simulink model "HLS_VMC_testing"  (R2025a)
settings: Solver=VariableStepAuto  StartTime=0.0  StopTime=0.0001  RelTol=1e-3
InitFcn:
  | fs = 500e6;
values from neighbouring files (symbols this model uses):
  N = length(X)    [outputPlots.m]
undefined symbols (not defined in the file or in its folder): A, es1, i, S, vsva2488, xcvr1602
libraries: hdlBasic x98, hlsBasic x64, aieUtilities x18, dspsrcs4 x15, dspxfrm3 x2, hdlDSPIP x2, hlsUtilities x1, vmcUtilities x1
(part 4 of 4)

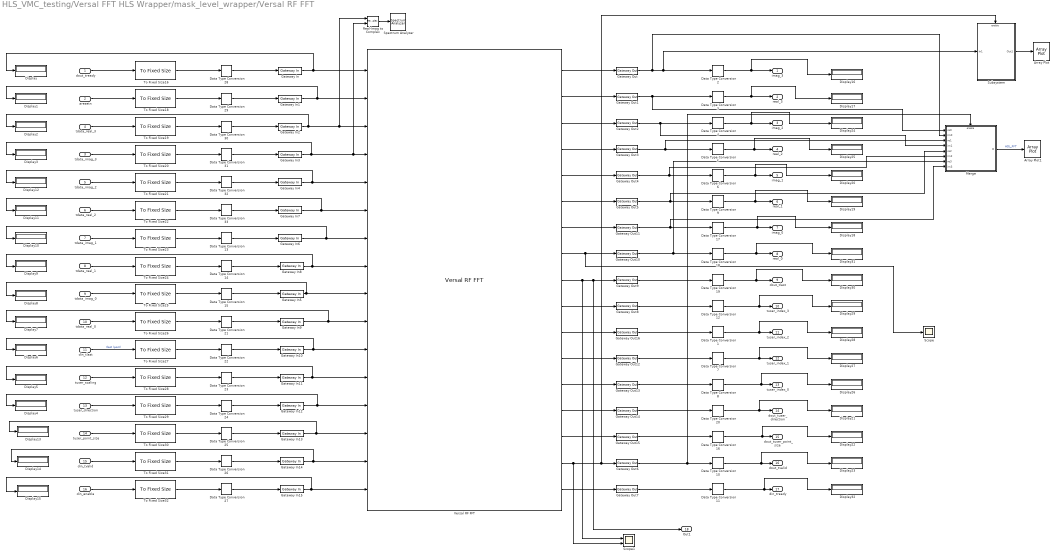
== system HLS_VMC_testing/Versal FFT HLS Wrapper/mask_level_wrapper/Versal RF FFT ==
  dout_tready : Inport
  aresetn : Inport  Port=2
  tdata_imag_3 : Inport  Port=3
  tdata_real_3 : Inport  Port=4
  tdata_imag_2 : Inport  Port=5
  tdata_real_2 : Inport  Port=6
  tdata_imag_1 : Inport  Port=7
  tdata_real_1 : Inport  Port=8
  tdata_imag_0 : Inport  Port=9
  tdata_real_0 : Inport  Port=10
  din_tlast : Inport  Port=11
  tuser_scaling : Inport  Port=12
  tuser_direction : Inport  Port=13
  tuser_point_size : Inport  Port=14
  din_tvalid : Inport  Port=15
  din_enable : Inport  Port=16
  Array Plot : ArrayPlot  WindowPosition=[880.000000,470.000000,800.000000,500.000000,]  ScopeFrameLocation=window  YLimits=[-10 10]
  Array Plot1 : ArrayPlot  WindowPosition=[880.000000,470.000000,800.000000,500.000000,]  ScopeFrameLocation=window  YLimits=[-10 10]
  Data Type Conversion{1,7..8,12} (4 alike) : hlsBasic/Data Type Conversion  OutDataType=data type expression  TypeExp='x_ufix12'  Signedness=Signed  WordLength=16  FractionalLength=0  RoundingMode=Truncation to minus infinity  OverflowMode=Wrap around
  Data Type Conversion{10..11,19..20} (4 alike) : hlsBasic/Data Type Conversion  OutDataType=data type expression  TypeExp='x_ufix1'  Signedness=Signed  WordLength=16  FractionalLength=0  RoundingMode=Truncation to minus infinity  OverflowMode=Wrap around
  Data Type Conversion{13..15,21..33} (16 alike) : hlsBasic/Data Type Conversion  OutDataType=double  TypeExp=''  Signedness=Signed  WordLength=16  FractionalLength=0  RoundingMode=Truncation to minus infinity  OverflowMode=Wrap around
  Data Type Conversion16 : hlsBasic/Data Type Conversion  OutDataType=data type expression  TypeExp='x_ufix4'  Signedness=Signed  WordLength=16  FractionalLength=0  RoundingMode=Truncation to minus infinity  OverflowMode=Wrap around
  Data Type Conversion{2..6,9,17..18} (8 alike) : hlsBasic/Data Type Conversion  OutDataType=data type expression  TypeExp='x_sfix16_En15'  Signedness=Signed  WordLength=16  FractionalLength=0  RoundingMode=Truncation to minus infinity  OverflowMode=Wrap around
  Display{,1..32} (33 alike) : Display
  Gateway In : hdlBasic/Gateway In  gui_display_data_type=Boolean  arith_type=Boolean  n_bits=16  bin_pt=15  preci_type=Single  exp_width=8  frac_width=24  rows=1  columns=1  quantization="Round  (unbiased: +/- Inf)"  overflow=Saturate  period=1/fs  UseAsADC=off  ADCChannel='1'  interface=None  automatic_assignment=on  address_offset=hex2dec('00')  intf_name=''  intf_description=''  default_value=0  timing_constraint=None  locs_specified=off  LOCs={}  io_standard={}  inherit_from_input=off  hdl_port=on  XmcBlockStatus=1  maskContainerNames=group4  block_type=gatewayin  block_config=sysgen:gateway_in_config  block_width_w=590  block_height_w=620  block_width=640  block_height=850
  Gateway In{1,10,14..15} (4 alike) : hdlBasic/Gateway In  gui_display_data_type=Boolean  arith_type=Boolean  n_bits=16  bin_pt=14  preci_type=Single  exp_width=8  frac_width=24  rows=1  columns=1  quantization="Round  (unbiased: +/- Inf)"  overflow=Saturate  period=1/fs  UseAsADC=off  ADCChannel='1'  interface=None  automatic_assignment=on  address_offset=hex2dec('00')  intf_name=''  intf_description=''  default_value=0  timing_constraint=None  locs_specified=off  LOCs={}  io_standard={}  inherit_from_input=off  hdl_port=on  XmcBlockStatus=1  maskContainerNames=group4  block_type=gatewayin  block_config=sysgen:gateway_in_config  block_width_w=590  block_height_w=620  block_width=640  block_height=850
  Gateway In11 : hdlBasic/Gateway In  gui_display_data_type=Fixed-point  arith_type=Unsigned  n_bits=13  bin_pt=13  preci_type=Single  exp_width=8  frac_width=24  rows=1  columns=1  quantization="Round  (unbiased: +/- Inf)"  overflow=Saturate  period=1/fs  UseAsADC=off  ADCChannel='1'  interface=None  automatic_assignment=on  address_offset=hex2dec('00')  intf_name=''  intf_description=''  default_value=0  timing_constraint=None  locs_specified=off  LOCs={}  io_standard={}  inherit_from_input=off  hdl_port=on  XmcBlockStatus=1  maskContainerNames=group4  block_type=gatewayin  block_config=sysgen:gateway_in_config  block_width_w=590  block_height_w=620  block_width=640  block_height=850
  Gateway In12 : hdlBasic/Gateway In  gui_display_data_type=Fixed-point  arith_type=Unsigned  n_bits=1  bin_pt=0  preci_type=Single  exp_width=8  frac_width=24  rows=1  columns=1  quantization="Round  (unbiased: +/- Inf)"  overflow=Saturate  period=1/fs  UseAsADC=off  ADCChannel='1'  interface=None  automatic_assignment=on  address_offset=hex2dec('00')  intf_name=''  intf_description=''  default_value=0  timing_constraint=None  locs_specified=off  LOCs={}  io_standard={}  inherit_from_input=off  hdl_port=on  XmcBlockStatus=1  maskContainerNames=group4  block_type=gatewayin  block_config=sysgen:gateway_in_config  block_width_w=590  block_height_w=620  block_width=640  block_height=850
  Gateway In13 : hdlBasic/Gateway In  gui_display_data_type=Fixed-point  arith_type=Unsigned  n_bits=4  bin_pt=0  preci_type=Single  exp_width=8  frac_width=24  rows=1  columns=1  quantization="Round  (unbiased: +/- Inf)"  overflow=Saturate  period=1/fs  UseAsADC=off  ADCChannel='1'  interface=None  automatic_assignment=on  address_offset=hex2dec('00')  intf_name=''  intf_description=''  default_value=0  timing_constraint=None  locs_specified=off  LOCs={}  io_standard={}  inherit_from_input=off  hdl_port=on  XmcBlockStatus=1  maskContainerNames=group4  block_type=gatewayin  block_config=sysgen:gateway_in_config  block_width_w=590  block_height_w=620  block_width=640  block_height=850
  Gateway In{2..9} (8 alike) : hdlBasic/Gateway In  gui_display_data_type=Fixed-point  arith_type=Signed (2's comp)  n_bits=18  bin_pt=17  preci_type=Single  exp_width=8  frac_width=24  rows=1  columns=1  quantization="Round  (unbiased: +/- Inf)"  overflow=Saturate  period=1/fs  UseAsADC=off  ADCChannel='1'  interface=None  automatic_assignment=on  address_offset=hex2dec('00')  intf_name=''  intf_description=''  default_value=0  timing_constraint=None  locs_specified=off  LOCs={}  io_standard={}  inherit_from_input=off  hdl_port=on  XmcBlockStatus=1  maskContainerNames=group4  block_type=gatewayin  block_config=sysgen:gateway_in_config  block_width_w=590  block_height_w=620  block_width=640  block_height=850
  Gateway Out{,1..16} (17 alike) : hdlBasic/Gateway Out  inherit_from_input=off  bool_to_boolean=off  hdl_port=on  rows=1  columns=1  UseAsDAC=off  DACChannel='1'  interface=None  automatic_assignment=on  address_offset=hex2dec('00')  intf_name=''  intf_description=''  timing_constraint=None  locs_specified=off  LOCs={}  io_standard={}  XmcBlockStatus=1  maskContainerNames=group4  block_type=gatewayout  block_config=sysgen:gateway_out_config  block_width_w=590  block_height_w=620  block_width=620  block_height=750
  Merge : Subsystem
  Real-Imag to Complex : RealImagToComplex
  Scope : Scope
      settings: ActiveDisplayYMinimum=-1  ActiveDisplayYMaximum=1  DataLoggingVariableName=ScopeData10
  Scope1 : Scope  NumInputPorts=2
      settings: ActiveDisplayYMinimum=-1  ActiveDisplayYMaximum=1  DataLoggingVariableName=ScopeData9
  Spectrum Analyzer : SpectrumAnalyzer  WindowPosition=[591.000000,490.000000,800.000000,500.000000,]  ScopeFrameLocation=window  WindowInvariantSamplesPerUpdate=on  YLimits=[-31.4263 39.9556]
  Subsystem : Subsystem
  To Fixed Size{16,18..32} (16 alike) : aieUtilities/To Fixed Size  Mode=Stop simulation when input variable-size signal is not full  OutputSize=Inherit: Same as input  CopyMethod=Buffer samples to form output  HasStatusOutput=on
  Versal RF FFT : hdlDSPIP/Versal RF FFT  sample_rate=4  fft_max_point_size_temp=1024  fft_max_point_size=10  fft_scaling=on  fft_reorder=on  events=off  ip_name=Versal RF FFT  enable_all_ports=false  mode=Streaming FFT  ip_version=1.1  dsptool_ready=false  ipcore_usecache=true  ipcore_useipmodelcache=true  wrapper_available=true  port_translation_map={ 'S_AXIS_aclken' => 'en', 'aresetn' => 'rst' }  structural_sim=true  ipcore_do_not_force_period=true  XmcBlockStatus=1  maskContainerNames=tabcontainer1  block_type=vrf_fft_v1_0  block_config=sysgen:rodinimport_config
  imag_3 : Outport
  real_3 : Outport  Port=2
  imag_2 : Outport  Port=3
  real_2 : Outport  Port=4
  imag_1 : Outport  Port=5
  real_1 : Outport  Port=6
  imag_0 : Outport  Port=7
  real_0 : Outport  Port=8
  dout_tlast : Outport  Port=9
  tuser_index_3 : Outport  Port=10
  tuser_index_2 : Outport  Port=11
  tuser_index_1 : Outport  Port=12
  tuser_index_0 : Outport  Port=13
  dout_tuser_direction : Outport  Port=14
  dout_tuser_point_size : Outport  Port=15
  dout_tvalid : Outport  Port=16
  din_tready : Outport  Port=17
  Out1 : Outport  Port=18
  wires:
  dout_tready/1 -> To Fixed Size16/1
  aresetn/1 -> To Fixed Size18/1
  tuser_point_size/1 -> To Fixed Size30/1
  tuser_direction/1 -> To Fixed Size29/1
  tuser_scaling/1 -> To Fixed Size28/1
  din_tlast/1 -> To Fixed Size27/1  "tlast (post)"
  din_tvalid/1 -> To Fixed Size31/1
  tdata_real_3/1 -> To Fixed Size19/1
  tdata_real_0/1 -> To Fixed Size26/1
  tdata_real_2/1 -> To Fixed Size22/1
  tdata_real_1/1 -> To Fixed Size24/1
  tdata_imag_0/1 -> To Fixed Size25/1
  tdata_imag_1/1 -> To Fixed Size23/1
  tdata_imag_2/1 -> To Fixed Size21/1
  tdata_imag_3/1 -> To Fixed Size20/1
  din_enable/1 -> To Fixed Size32/1
  Versal RF FFT/2 -> Gateway Out1/1
  Versal RF FFT/3 -> Gateway Out2/1
  Versal RF FFT/4 -> Gateway Out3/1
  Versal RF FFT/5 -> Gateway Out4/1
  Versal RF FFT/6 -> Gateway Out5/1
  Versal RF FFT/7 -> Gateway Out11/1
  Versal RF FFT/8 -> Scope/1, Gateway Out10/1
  Versal RF FFT/10 -> Gateway Out8/1
  Versal RF FFT/11 -> Gateway Out16/1
  Versal RF FFT/1 -> Gateway Out/1
  To Fixed Size16/1 -> Data Type Conversion28/1
  To Fixed Size18/1 -> Data Type Conversion29/1
  To Fixed Size19/1 -> Data Type Conversion30/1
  To Fixed Size20/1 -> Data Type Conversion31/1
  To Fixed Size21/1 -> Data Type Conversion32/1
  To Fixed Size22/1 -> Data Type Conversion33/1
  To Fixed Size23/1 -> Data Type Conversion13/1
  To Fixed Size24/1 -> Data Type Conversion14/1
  To Fixed Size25/1 -> Data Type Conversion15/1
  To Fixed Size26/1 -> Data Type Conversion21/1
  To Fixed Size27/1 -> Data Type Conversion22/1
  To Fixed Size28/1 -> Data Type Conversion23/1
  To Fixed Size29/1 -> Data Type Conversion24/1
  To Fixed Size30/1 -> Data Type Conversion25/1
  To Fixed Size31/1 -> Data Type Conversion26/1
  To Fixed Size32/1 -> Data Type Conversion27/1
  Gateway In/1 -> Display/1, Versal RF FFT/1
  Gateway In1/1 -> Display1/1, Versal RF FFT/2
  Gateway In4/1 -> Display12/1, Versal RF FFT/5
  Gateway In7/1 -> Display11/1, Versal RF FFT/6
  Gateway In6/1 -> Display10/1, Versal RF FFT/7
  Gateway In9/1 -> Display7/1, Versal RF FFT/10
  Gateway In5/1 -> Display8/1, Versal RF FFT/9
  Gateway In10/1 -> Display6/1, Versal RF FFT/11
  Gateway In11/1 -> Display5/1, Versal RF FFT/12
  Gateway Out1/1 -> Merge/1(re0), Data Type Conversion3/1
  Gateway Out2/1 -> Merge/4(im1), Data Type Conversion4/1
  Gateway Out3/1 -> Merge/3(re1), Data Type Conversion5/1
  Gateway Out4/1 -> Merge/6(im2), Data Type Conversion6/1
  Gateway Out5/1 -> Merge/5(re2), Data Type Conversion9/1
  Gateway Out11/1 -> Merge/8(im3), Data Type Conversion17/1
  Gateway Out10/1 -> Merge/7(re3), Data Type Conversion18/1
  Gateway Out9/1 -> Data Type Conversion19/1
  Gateway Out6/1 -> Merge/Enable, Data Type Conversion10/1
  Gateway Out7/1 -> Data Type Conversion11/1
  Gateway Out8/1 -> Data Type Conversion12/1
  Gateway Out16/1 -> Data Type Conversion1/1
  Gateway Out12/1 -> Data Type Conversion7/1
  Gateway Out13/1 -> Data Type Conversion8/1
  Gateway Out15/1 -> Data Type Conversion16/1
  Gateway Out14/1 -> Data Type Conversion20/1
  Data Type Conversion2/1 -> Display16/1, imag_3/1
  Data Type Conversion3/1 -> Display17/1, real_3/1
  Data Type Conversion4/1 -> Display24/1, imag_2/1
  Data Type Conversion5/1 -> Display25/1, real_2/1
  Data Type Conversion6/1 -> Display20/1, imag_1/1
  Data Type Conversion9/1 -> Display19/1, real_1/1
  Data Type Conversion17/1 -> Display18/1, imag_0/1
  Data Type Conversion19/1 -> Display30/1, dout_tlast/1
  Data Type Conversion12/1 -> Display29/1, tuser_index_3/1
  Data Type Conversion1/1 -> Display28/1, tuser_index_2/1
  Data Type Conversion7/1 -> Display27/1, tuser_index_1/1
  Data Type Conversion8/1 -> Display26/1, tuser_index_0/1
  Data Type Conversion20/1 -> Display21/1, dout_tuser_direction/1
  Data Type Conversion16/1 -> Display22/1, dout_tuser_point_size/1
  Data Type Conversion10/1 -> Display23/1, dout_tvalid/1
  Data Type Conversion11/1 -> Display32/1, din_tready/1
  Versal RF FFT/9 -> Scope1/1, Out1/1, Gateway Out9/1
  Gateway In12/1 -> Display4/1, Versal RF FFT/13
  Gateway In14/1 -> Display14/1, Versal RF FFT/15
  Gateway In15/1 -> Display15/1, Versal RF FFT/16
  Gateway In13/1 -> Display13/1, Versal RF FFT/14
  Versal RF FFT/12 -> Gateway Out12/1
  Versal RF FFT/13 -> Gateway Out13/1
  Versal RF FFT/14 -> Gateway Out14/1
  Versal RF FFT/15 -> Gateway Out15/1
  Versal RF FFT/16 -> Scope1/2, Subsystem/Enable, Gateway Out6/1
  Versal RF FFT/17 -> Gateway Out7/1
  Data Type Conversion28/1 -> Gateway In/1
  Data Type Conversion29/1 -> Gateway In1/1
  Data Type Conversion30/1 -> Gateway In2/1
  Data Type Conversion31/1 -> Gateway In3/1
  Data Type Conversion32/1 -> Gateway In4/1
  Data Type Conversion33/1 -> Gateway In7/1
  Data Type Conversion13/1 -> Gateway In6/1
  Data Type Conversion14/1 -> Gateway In8/1
  Data Type Conversion15/1 -> Gateway In5/1
  Data Type Conversion21/1 -> Gateway In9/1
  Data Type Conversion22/1 -> Gateway In10/1
  Data Type Conversion23/1 -> Gateway In11/1
  Data Type Conversion24/1 -> Gateway In12/1
  Data Type Conversion25/1 -> Gateway In13/1
  Data Type Conversion26/1 -> Gateway In14/1
  Data Type Conversion27/1 -> Gateway In15/1
  Gateway In8/1 -> Display9/1, Versal RF FFT/8
  Data Type Conversion18/1 -> Display31/1, real_0/1
  Gateway In2/1 -> Display2/1, Real-Imag to Complex/1, Versal RF FFT/3
  Gateway In3/1 -> Display3/1, Real-Imag to Complex/2, Versal RF FFT/4
  Real-Imag to Complex/1 -> Spectrum Analyzer/1
  Gateway Out/1 -> Merge/2(im0), Subsystem/1(In1), Data Type Conversion2/1
  Subsystem/1(Out1) -> Array Plot/1
  Merge/1(O) -> Array Plot1/1  "HDL_FFT"

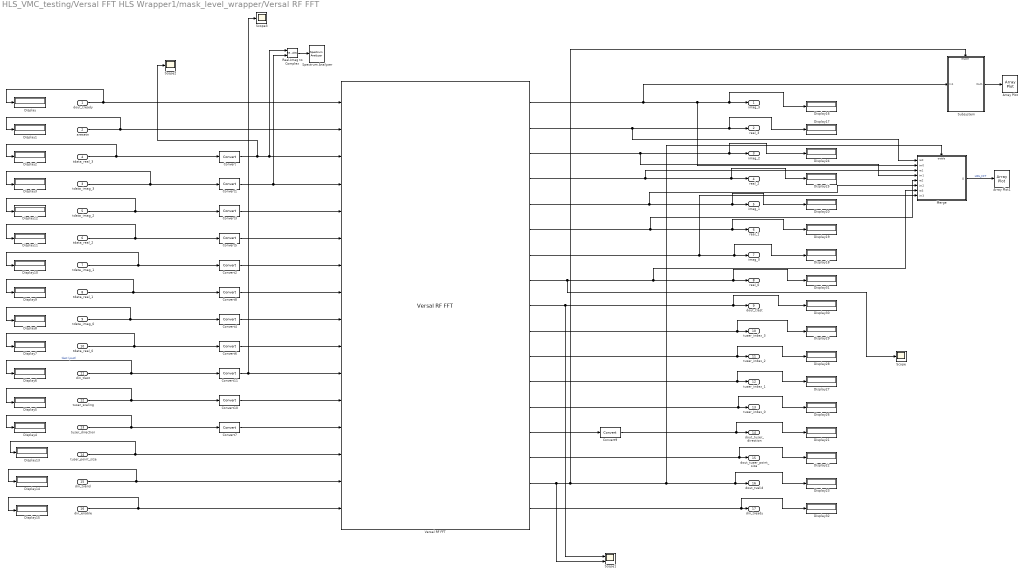
== system HLS_VMC_testing/Versal FFT HLS Wrapper1/mask_level_wrapper/Versal RF FFT ==
  dout_tready : Inport
  aresetn : Inport  Port=2
  tdata_imag_3 : Inport  Port=3
  tdata_real_3 : Inport  Port=4
  tdata_imag_2 : Inport  Port=5
  tdata_real_2 : Inport  Port=6
  tdata_imag_1 : Inport  Port=7
  tdata_real_1 : Inport  Port=8
  tdata_imag_0 : Inport  Port=9
  tdata_real_0 : Inport  Port=10
  din_tlast : Inport  Port=11
  tuser_scaling : Inport  Port=12
  tuser_direction : Inport  Port=13
  tuser_point_size : Inport  Port=14
  din_tvalid : Inport  Port=15
  din_enable : Inport  Port=16
  Array Plot : ArrayPlot  WindowPosition=[1.000000,1.000000,2560.000000,1389.000000,]  ScopeFrameLocation=window  YLimits=[-10 10]
  Array Plot1 : ArrayPlot  WindowPosition=[1.000000,1.000000,2560.000000,1389.000000,]  ScopeFrameLocation=window  YLimits=[-10 10]
  Convert{,1..6,8} (8 alike) : hdlBasic/Convert  gui_display_data_type=Fixed-point  arith_type="Signed  (2's comp)"  n_bits=18  bin_pt=17  float_type=Single  exp_bits=8  fraction_bits=24  quantization=Truncate  overflow=Wrap  en=off  latency=0  pipeline=off  XmcBlockStatus=1  maskContainerNames=group2  block_type=convert  block_config=sysgen:Convert_config  block_width=595  block_height=885
  Convert10 : hdlBasic/Convert  gui_display_data_type=Fixed-point  arith_type=Unsigned  n_bits=13  bin_pt=13  float_type=Single  exp_bits=8  fraction_bits=24  quantization=Truncate  overflow=Wrap  en=off  latency=0  pipeline=off  XmcBlockStatus=1  maskContainerNames=group2  block_type=convert  block_config=sysgen:Convert_config  block_width=595  block_height=885
  Convert11 : hdlBasic/Convert  gui_display_data_type=Boolean  arith_type=Boolean  n_bits=18  bin_pt=17  float_type=Single  exp_bits=8  fraction_bits=24  quantization=Truncate  overflow=Wrap  en=off  latency=0  pipeline=off  XmcBlockStatus=1  maskContainerNames=group2  block_type=convert  block_config=sysgen:Convert_config  block_width=595  block_height=885
  Convert7 : hdlBasic/Convert  gui_display_data_type=Fixed-point  arith_type=Unsigned  n_bits=1  bin_pt=0  float_type=Single  exp_bits=8  fraction_bits=24  quantization=Truncate  overflow=Wrap  en=off  latency=0  pipeline=off  XmcBlockStatus=1  maskContainerNames=group2  block_type=convert  block_config=sysgen:Convert_config  block_width=595  block_height=885
  Convert9 : hdlBasic/Convert  gui_display_data_type=Boolean  arith_type=Boolean  n_bits=1  bin_pt=0  float_type=Single  exp_bits=8  fraction_bits=24  quantization=Truncate  overflow=Wrap  en=off  latency=0  pipeline=off  XmcBlockStatus=1  maskContainerNames=group2  block_type=convert  block_config=sysgen:Convert_config  block_width=595  block_height=885
  Display{,1..32} (33 alike) : Display
  Merge : Subsystem
  Real-Imag to Complex : RealImagToComplex
  Scope : Scope
      settings: ActiveDisplayYMinimum=-1  ActiveDisplayYMaximum=1  DataLoggingVariableName=ScopeData10
  Scope1 : Scope  NumInputPorts=2
      settings: ActiveDisplayYMinimum=-1  ActiveDisplayYMaximum=1  DataLoggingVariableName=ScopeData9
  Scope2 : Scope
      settings: ActiveDisplayYMinimum=-1  ActiveDisplayYMaximum=1  DataLoggingVariableName=ScopeData22
  Scope3 : Scope
      settings: ActiveDisplayYMinimum=-1  ActiveDisplayYMaximum=1  DataLoggingVariableName=ScopeData23
  Spectrum Analyzer : SpectrumAnalyzer  WindowPosition=[880.000000,470.000000,800.000000,500.000000,]  ScopeFrameLocation=window  WindowInvariantSamplesPerUpdate=on  Span=499999999.99999994  StartFrequency=-249999999.99999997  StopFrequency=249999999.99999997  YLimits=[-46.6022 38.4581]
  Subsystem : Subsystem
  Versal RF FFT : hdlDSPIP/Versal RF FFT  sample_rate=4  fft_max_point_size_temp=1024  fft_max_point_size=10  fft_scaling=on  fft_reorder=on  events=off  ip_name=Versal RF FFT  enable_all_ports=false  mode=Streaming FFT  ip_version=1.1  dsptool_ready=false  ipcore_usecache=true  ipcore_useipmodelcache=true  wrapper_available=true  port_translation_map={ 'S_AXIS_aclken' => 'en', 'aresetn' => 'rst' }  structural_sim=true  ipcore_do_not_force_period=true  XmcBlockStatus=1  maskContainerNames=tabcontainer1  block_type=vrf_fft_v1_0  block_config=sysgen:rodinimport_config
  imag_3 : Outport
  real_3 : Outport  Port=2
  imag_2 : Outport  Port=3
  real_2 : Outport  Port=4
  imag_1 : Outport  Port=5
  real_1 : Outport  Port=6
  imag_0 : Outport  Port=7
  real_0 : Outport  Port=8
  dout_tlast : Outport  Port=9
  tuser_index_3 : Outport  Port=10
  tuser_index_2 : Outport  Port=11
  tuser_index_1 : Outport  Port=12
  tuser_index_0 : Outport  Port=13
  dout_tuser_direction : Outport  Port=14
  dout_tuser_point_size : Outport  Port=15
  dout_tvalid : Outport  Port=16
  din_tready : Outport  Port=17
  wires:
  aresetn/1 -> Display1/1, Versal RF FFT/2
  din_tlast/1 -> Display6/1, Convert11/1  "tlast (post)"
  tdata_imag_2/1 -> Display12/1, Convert3/1
  tdata_imag_1/1 -> Display10/1, Convert2/1
  tdata_real_0/1 -> Display7/1, Convert6/1
  tdata_imag_0/1 -> Display8/1, Convert4/1
  Versal RF FFT/1 -> Merge/2(im0), Display16/1, imag_3/1, Subsystem/1(In1)
  Versal RF FFT/2 -> Display17/1, real_3/1, Merge/1(re0)
  Versal RF FFT/3 -> Display24/1, imag_2/1, Merge/4(im1)
  Versal RF FFT/4 -> Display25/1, real_2/1, Merge/3(re1)
  Versal RF FFT/5 -> Display20/1, imag_1/1, Merge/6(im2)
  Versal RF FFT/6 -> Display19/1, real_1/1, Merge/5(re2)
  Versal RF FFT/7 -> Display18/1, imag_0/1, Merge/8(im3)
  Versal RF FFT/9 -> Scope1/1, Display30/1, dout_tlast/1
  Versal RF FFT/10 -> Display29/1, tuser_index_3/1
  Versal RF FFT/11 -> Display28/1, tuser_index_2/1
  Versal RF FFT/12 -> Display27/1, tuser_index_1/1
  Versal RF FFT/13 -> Display26/1, tuser_index_0/1
  Versal RF FFT/14 -> Convert9/1
  Versal RF FFT/15 -> Display22/1, dout_tuser_point_size/1
  Versal RF FFT/16 -> Scope1/2, Merge/Enable, Display23/1, dout_tvalid/1, Subsystem/Enable
  Versal RF FFT/17 -> Display32/1, din_tready/1
  tdata_real_1/1 -> Display9/1, Convert8/1
  Versal RF FFT/8 -> Display31/1, real_0/1, Merge/7(re3), Scope/1
  tdata_real_3/1 -> Display2/1, Convert/1
  Real-Imag to Complex/1 -> Spectrum Analyzer/1
  Subsystem/1(Out1) -> Array Plot/1
  Merge/1(O) -> Array Plot1/1  "HDL_FFT"
  tuser_scaling/1 -> Display5/1, Convert10/1
  tuser_direction/1 -> Display4/1, Convert7/1
  tuser_point_size/1 -> Display13/1, Versal RF FFT/14
  din_tvalid/1 -> Display14/1, Versal RF FFT/15
  din_enable/1 -> Display15/1, Versal RF FFT/16
  dout_tready/1 -> Display/1, Versal RF FFT/1
  tdata_imag_3/1 -> Display3/1, Convert1/1
  tdata_real_2/1 -> Display11/1, Convert5/1
  Convert/1 -> Scope2/1, Versal RF FFT/3, Real-Imag to Complex/1
  Convert3/1 -> Versal RF FFT/5
  Convert1/1 -> Versal RF FFT/4, Real-Imag to Complex/2
  Convert5/1 -> Versal RF FFT/6
  Convert2/1 -> Versal RF FFT/7
  Convert8/1 -> Versal RF FFT/8
  Convert4/1 -> Versal RF FFT/9
  Convert6/1 -> Versal RF FFT/10
  Convert7/1 -> Versal RF FFT/13
  Convert10/1 -> Versal RF FFT/12
  Convert9/1 -> Display21/1, dout_tuser_direction/1
  Convert11/1 -> Versal RF FFT/11, Scope3/1

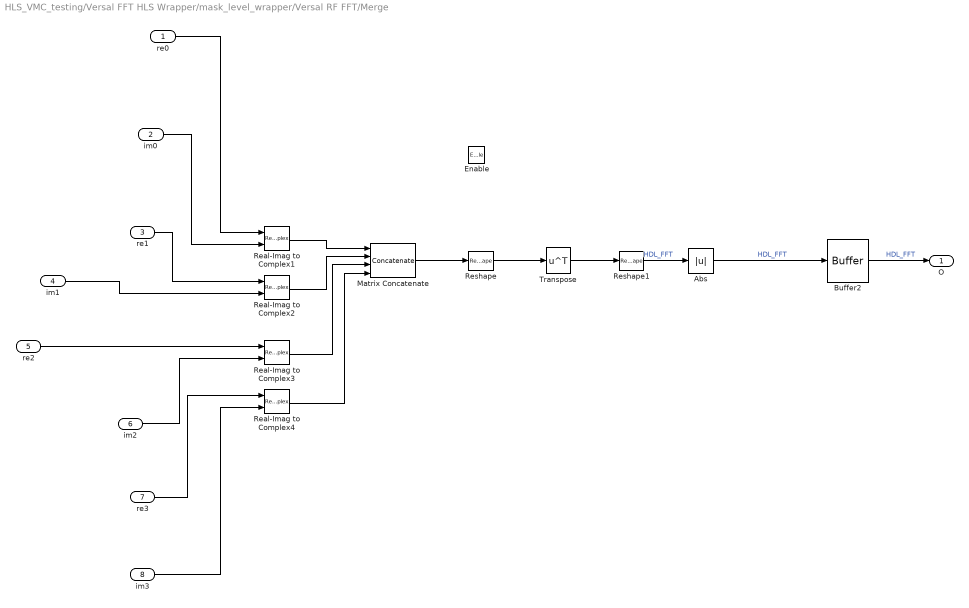
== system HLS_VMC_testing/Versal FFT HLS Wrapper/mask_level_wrapper/Versal RF FFT/Merge ==
  re0 : Inport
  im0 : Inport  Port=2
  re1 : Inport  Port=3
  im1 : Inport  Port=4
  re2 : Inport  Port=5
  im2 : Inport  Port=6
  re3 : Inport  Port=7
  im3 : Inport  Port=8
  Enable : EnablePort
  Abs : Abs  SaturateOnIntegerOverflow=off
  Buffer2 : Buffer  N=1024  OutputFrames=off
  Matrix Concatenate : Concatenate  NumInputs=4  Mode=Multidimensional array
  Real-Imag to Complex{1..4} (4 alike) : RealImagToComplex
  Reshape : Reshape  OutputDimensionality=Customize  OutputDimensions=[1, 4]
  Reshape1 : Reshape  OutputDimensions=[1, 10]
  Transpose : Math  Operator=transpose
  O : Outport
  wires:
  Reshape1/1 -> Abs/1  "HDL_FFT"
  Abs/1 -> Buffer2/1  "HDL_FFT"
  Buffer2/1 -> O/1  "HDL_FFT"
  im0/1 -> Real-Imag to Complex1/2
  re0/1 -> Real-Imag to Complex1/1
  im1/1 -> Real-Imag to Complex2/2
  re1/1 -> Real-Imag to Complex2/1
  Real-Imag to Complex1/1 -> Matrix Concatenate/1
  Real-Imag to Complex2/1 -> Matrix Concatenate/2
  Transpose/1 -> Reshape1/1
  Reshape/1 -> Transpose/1
  Matrix Concatenate/1 -> Reshape/1
  re2/1 -> Real-Imag to Complex3/1
  im2/1 -> Real-Imag to Complex3/2
  re3/1 -> Real-Imag to Complex4/1
  Real-Imag to Complex4/1 -> Matrix Concatenate/4
  Real-Imag to Complex3/1 -> Matrix Concatenate/3
  im3/1 -> Real-Imag to Complex4/2

== system HLS_VMC_testing/Versal FFT HLS Wrapper/mask_level_wrapper/Versal RF FFT/Subsystem ==
  In1 : Inport
  Enable : EnablePort
  Abs : Abs  SaturateOnIntegerOverflow=off
  Buffer : Buffer  N=1024  OutputFrames=off
  Out1 : Outport
  wires:
  In1/1 -> Abs/1
  Buffer/1 -> Out1/1
  Abs/1 -> Buffer/1

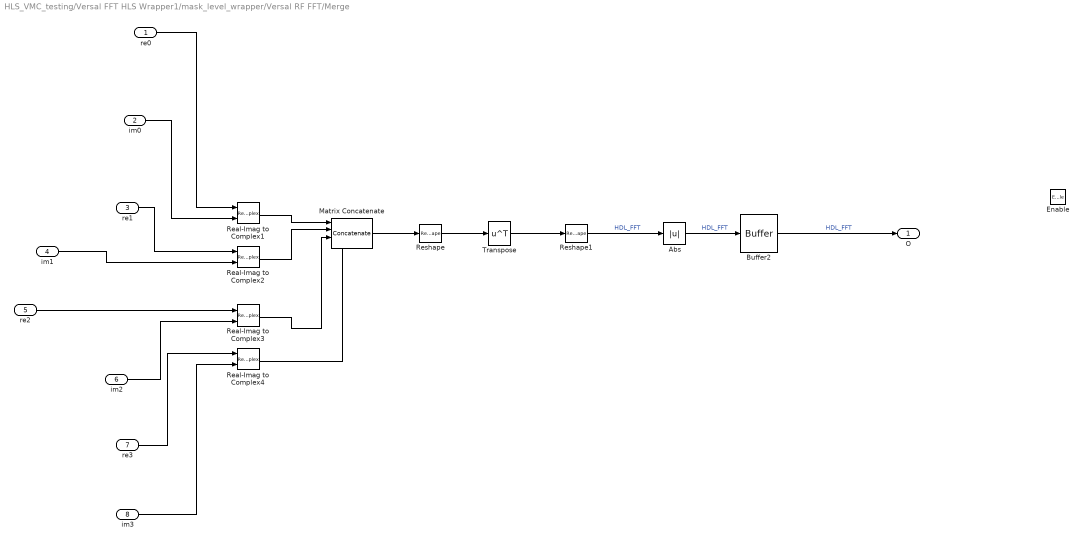
== system HLS_VMC_testing/Versal FFT HLS Wrapper1/mask_level_wrapper/Versal RF FFT/Merge ==
  re0 : Inport
  im0 : Inport  Port=2
  re1 : Inport  Port=3
  im1 : Inport  Port=4
  re2 : Inport  Port=5
  im2 : Inport  Port=6
  re3 : Inport  Port=7
  im3 : Inport  Port=8
  Enable : EnablePort
  Abs : Abs  SaturateOnIntegerOverflow=off
  Buffer2 : Buffer  N=1024  OutputFrames=off
  Matrix Concatenate : Concatenate  NumInputs=4  Mode=Multidimensional array
  Real-Imag to Complex{1..4} (4 alike) : RealImagToComplex
  Reshape : Reshape  OutputDimensionality=Customize  OutputDimensions=[1, 4]
  Reshape1 : Reshape  OutputDimensions=[1, 10]
  Transpose : Math  Operator=transpose
  O : Outport
  wires:
  Reshape1/1 -> Abs/1  "HDL_FFT"
  Abs/1 -> Buffer2/1  "HDL_FFT"
  Buffer2/1 -> O/1  "HDL_FFT"
  im0/1 -> Real-Imag to Complex1/2
  re0/1 -> Real-Imag to Complex1/1
  im1/1 -> Real-Imag to Complex2/2
  re1/1 -> Real-Imag to Complex2/1
  Real-Imag to Complex1/1 -> Matrix Concatenate/1
  Real-Imag to Complex2/1 -> Matrix Concatenate/2
  Transpose/1 -> Reshape1/1
  Reshape/1 -> Transpose/1
  Matrix Concatenate/1 -> Reshape/1
  re2/1 -> Real-Imag to Complex3/1
  im2/1 -> Real-Imag to Complex3/2
  re3/1 -> Real-Imag to Complex4/1
  Real-Imag to Complex4/1 -> Matrix Concatenate/4
  Real-Imag to Complex3/1 -> Matrix Concatenate/3
  im3/1 -> Real-Imag to Complex4/2

== system HLS_VMC_testing/Versal FFT HLS Wrapper1/mask_level_wrapper/Versal RF FFT/Subsystem ==
  In1 : Inport
  Enable : EnablePort
  Abs : Abs  SaturateOnIntegerOverflow=off
  Buffer : Buffer  N=1024  OutputFrames=off
  Display : Display
  Out1 : Outport
  wires:
  In1/1 -> Abs/1
  Buffer/1 -> Display/1, Out1/1
  Abs/1 -> Buffer/1
